simulink model "elec_thermal_mosfet_characteristics_model"  (R2017a)
settings: Solver=VariableStepAuto  StartTime=0.0  StopTime=SimTime  RelTol=1e-3  AbsTol=1e-3  EnableMultiTasking=on
model workspace (MAT data in the model file):
  SimTime = 10
  alpha = 0
  beta = 5
  cgdo = 55
  cgso = 255
  cj0 = 150
  cox = 410
  etabet = 1.3
  etais = 3
  etar = 0.95
  etasat = 1.04
  gamma = 0.5
  is = 1e-09
  m = 8
  n = 1
  phib = 0.95
  rca = 1
  rd = 0.01
  rg = 0.001
  rjc = 1
  rs = 0.0001
  stphib = -0.00085
  stvfb = 0.0005
  t0c = 25
  t0j = 25
  tDrain = [0 10]
  tGate = [0 10]
  tSource = [0 10]
  tamb = 85
  tauc = 500
  tauj = 500
  thesat = 0
  tmeas = 25
  tt = 50
  vDrain = [0 20]
  vGate = [1.5 1.5]
  vSource = [0 0]
  vfb = -1.05
  vj = 0.6
  vp = 0.05
libraries: fl_lib x5, elec_lib x4, nesl_utility x2
Description:
  | This test model is used by the elec_thermal_mosfet_characteristics app. It is invoked by the
  | app when generating current-voltage and capacitance-voltage characteristics.
  | 
  | 
  | Copyright 2016-2017 The MathWorks, Inc.
settings Model: Creator=MathWorks  LastModifiedBy=Discovery
settings DebuggingCC: SFUnexpectedBacktrackingDiag=warning  SFNoUnconditionalDefaultTransitionDiag=warning  SFExecutionAtInitializationDiag=none
settings GRTTargetCC: TargetLangStandard=C89/C90 (ANSI)
settings ConfigComp: CovMetricSettings=dw  CovHtmlReporting=on  CovSaveCumulativeToWorkspaceVar=on  CovSaveSingleToWorkspaceVar=on  CovShowResultsExplorer=off  CovExternalEMLEnable=off
settings SimscapeCC: SimscapeLogType=all  SimscapeLogName=simlog_elec_thermal_mosfet_characteristics  SimscapeLogLimitData=off  SimscapeLogDataHistory=10000

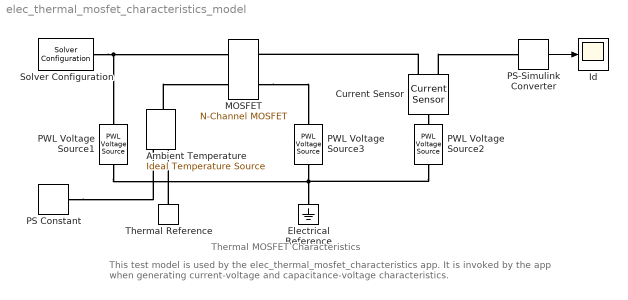
== system elec_thermal_mosfet_characteristics_model ==
  note: This test model is used by the elec_thermal_mosfet_characteristics app. It is invoked by the app when generating current-voltage and capacitance-voltage characteristics.
  note: Thermal MOSFET Characteristics
  Ambient Temperature : fl_lib/Thermal/Thermal Sources/Ideal Temperature Source
      settings: SourceProductName=Simscape  SourceProductBaseCode=SS
  Current Sensor : fl_lib/Electrical/Electrical Sensors/Current Sensor
  Electrical Reference : fl_lib/Electrical/Electrical Elements/Electrical Reference
  Id : Scope
  MOSFET : elec_lib/Semiconductor Devices/N-Channel MOSFET  parameterization=1  prmDatasheet=1  prmEquCoeff=1  Beta=5 A/V^2  Rds=0.025 Ohm  Id=6 A  Vgs=10 V  Vth=1.7 V  lam=0 1/V  Tmeas=25 degC  RS=1e-4 Ohm  RD=0.01 Ohm  C_param=1  C_GS=270 pF  C_GD=80 pF  C_DS=0 pF  C_iss=350 pF  C_rss=80 pF  C_oss=0 pF  C_GS_vec=[ 270 300 290 280 295 255 ] pF  C_GD_vec=[ 450 400 300 190 95 55 ] pF  C_DS_vec=[ 450 410 390 230 175 115 ] pF  C_iss_vec=[ 720 700 590 470 390 310 ] pF  C_rss_vec=[ 450 400 300 190 95 55 ] pF  C_oss_vec=[ 900 810 690 420 270 170 ] pF  C_Vds_vec=[ 0.1 0.3 1 3 10 30 ] V  V_GS_for_cap_data=0 V  charge_linearity_param=1  C_OX=200 pF  V_C_OX=-0.5 V  IsDiode=0 A  Vbi=vj V  n=n  Cj0Diode=0 pF  TT=tt ns  dVth_dT=-6 mV/K  Rds_T2=0.037 Ohm  Tmeas2=125 degC  BEXDatasheet=-1.5  BEXEquCoeff=-1.5  etaisDatasheet=3  etaisEquCoeff=3  TdeviceDatasheet=25 degC  TdeviceEquCoeff=25 degC  Rth=[rjc rca] K/W  thermal_mass_parameterization=1  thermal_mass=[tauj/rjc tauc/rca] J/K  thermal_time_constant=[tauj tauc] ns  thermal_mass_initial_temperatures=[ 25 25 ] degC  betaref=beta A/V^2  Vfbref=vfb V  gamma=gamma V^0.50000  phib2ref=phib V  thesatref=thesat 1/V  alpha=alpha  Vp=vp V  thesrref=0 1/V  m=m  Tref=tmeas degC  Cox=cox pF  Cgso=cgso pF  Cgdo=cgdo pF  Rsref=rs Ohm  Rdref=rd Ohm  Rgref=rg Ohm  Isref=is A  Cj0=cj0 pF  Tprm=1  etabet=etabet  Stvfb=stvfb V/K  Stphib=stphib V/K  etasat=etasat  etasr=0.65  etar=etar  etais=etais  Tsim=25 degC  T0=[t0j t0c] degC
      settings: SourceProductName=Simscape Electronics  SourceProductBaseCode=SN
  PS Constant : fl_lib/Physical Signals/Sources/PS Constant  constant=tamb+273.15
  PS-Simulink Converter : nesl_utility/PS-Simulink Converter  PhysicalDomain=network_engine_domain  SubClassName=ps_output  LeftPortType=input  RightPortType=output  PseudoPeriodic=off  Frequencies=[]  Unit=1  AffineConversion=off
  PWL Voltage Source1 : elec_lib/Additional Components/SPICE-Compatible Components/Sources/PWL Voltage Source  TIMElist=tGate s  VOLTlist=vGate V  INTERP=1  EXTRAP=2
      settings: SourceProductName=Simscape Electronics  SourceProductBaseCode=SN
  PWL Voltage Source2 : elec_lib/Additional Components/SPICE-Compatible Components/Sources/PWL Voltage Source  TIMElist=tDrain s  VOLTlist=vDrain V  INTERP=1  EXTRAP=2
      settings: SourceProductName=Simscape Electronics  SourceProductBaseCode=SN
  PWL Voltage Source3 : elec_lib/Additional Components/SPICE-Compatible Components/Sources/PWL Voltage Source  TIMElist=tSource s  VOLTlist=vSource V  INTERP=1  EXTRAP=2
      settings: SourceProductName=Simscape Electronics  SourceProductBaseCode=SN
  Solver Configuration : nesl_utility/Solver Configuration  PhysicalDomain=network_engine_domain  SubClassName=solver  LeftPortType=input  RightPortType=generic  Accelerate=off  Tones=[]  Harmonics=[]  SimulateNoise=off  Profile=off  UseLocalSampling=off  EnableSwitchedLinearOptims=on  FrequencyDomain=off  UseCCode=off  RelTol=0.001  AbsTol=1e-06  MinStep=1e-09  ToWorkspace=off  RevertToSquareIcSolve=off  NumHomotopyIterations=100  PhasorMode=off  PhasorModeNumHarmonics=1  OverrideAbsTol=off  DoDC=on  ResidualTolerance=1e-09  UseLocalSolver=off  LocalSolverChoice=NE_BACKWARD_EULER_ADVANCER  LocalSolverSampleTime=0.001  DoFixedCost=off  MaxNonlinIter=3  MaxModeIter=2  LinearAlgebra=Sparse  DelaysMemoryBudget=1024  AutomaticFiltering=on  FilteringTimeConstant=0.001
  Thermal Reference : fl_lib/Thermal/Thermal Elements/Thermal Reference
  wires:
  PS-Simulink Converter/1 -> Id/1
  connections:
  Solver Configuration/RConn1 -- MOSFET/LConn1 -- PWL Voltage Source1/LConn1
  MOSFET/RConn2 -- PWL Voltage Source3/LConn1
  PWL Voltage Source3/RConn1 -- PWL Voltage Source2/RConn1 -- Electrical Reference/LConn1 -- PWL Voltage Source1/RConn1
  Current Sensor/LConn1 -- PWL Voltage Source2/LConn1
  Current Sensor/RConn2 -- MOSFET/RConn1
  Current Sensor/RConn1 -- PS-Simulink Converter/LConn1
  Ambient Temperature/LConn1 -- MOSFET/LConn2
  Thermal Reference/LConn1 -- Ambient Temperature/RConn2
  PS Constant/RConn1 -- Ambient Temperature/RConn1
